simulink model "RoadBump"  (R2018b)
settings: Solver=VariableStepAuto  StartTime=0.0  StopTime=10  RelTol=1e-3
libraries: simulink x1
settings Model: Creator=oxyoung  LastModifiedBy=Administrator

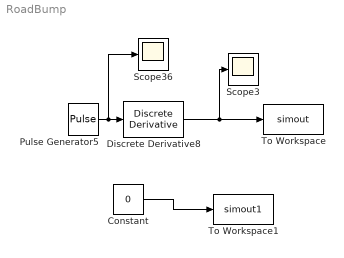
== system RoadBump ==
  Constant : Constant  Value=0
  Discrete Derivative8 : simulink/Quick Insert/Discrete/Discrete Derivative  gainval=1.0  ICPrevScaledInput=0.0  OutMin=[]  OutMax=[]  OutDataType=fixdt(1, 16)  OutScaling=2^-10  DoSatur=off
      settings: SourceProductName=Simulink  SourceProductBaseCode=SL
  Pulse Generator5 : DiscretePulseGenerator  PulseType=Time based  Amplitude=0.01  Period=1/0.3  PulseWidth=20
  Scope3 : Scope
  Scope36 : Scope
  To Workspace : ToWorkspace  VariableName=simout  SaveFormat=Structure With Time  SampleTime=0.002
  To Workspace1 : ToWorkspace  VariableName=simout1  SaveFormat=Structure With Time  SampleTime=0.002
  wires:
  Pulse Generator5/1 -> Scope36/1, Discrete Derivative8/1
  Discrete Derivative8/1 -> To Workspace/1, Scope3/1
  Constant/1 -> To Workspace1/1
